simulink model "slexDynamicSchedulingExample"  (R2019b)
settings: Solver=FixedStepAuto  StartTime=0.0  StopTime=1  FixedStep=1  RelTol=1e-3
libraries: simulink x2
settings Model: Creator=The MathWorks, Inc.  LastModifiedBy=bhisma
settings DataIOCC: SaveFormat=Array
settings OptimizationCC: DefaultParameterBehavior=Inlined  PassReuseOutputArgsThreshold=0
settings DebuggingCC: ParameterTunabilityLossMsg=error  ArithmeticOperatorsInVariantConditions=warning
settings SFSimCC: SimUseLocalCustomCode=off  MATLABDynamicMemAlloc=off  CustomCodeUndefinedFunction=UseInterfaceOnly
settings RTWCC: Description=Generic Real-Time Target  GenerateReport=on  RTWUseLocalCustomCode=off  LaunchReport=on
settings CodeAppCC: ForceParamTrailComments=on  OperatorAnnotations=on

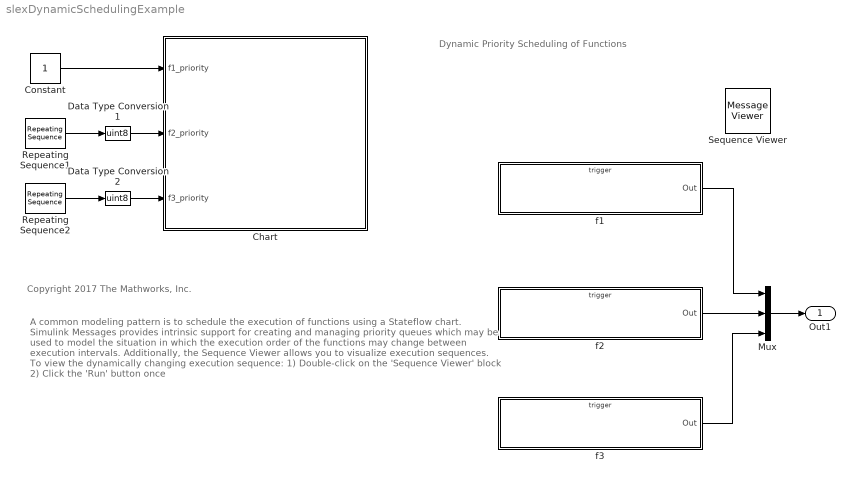
== system slexDynamicSchedulingExample ==
  note: A common modeling pattern is to schedule the execution of functions using a Stateflow chart. Simulink Messages provides intrinsic support for creating and managing priority queues which may be used to model the situation in which the execution order of the functions may change between execution intervals.
      |
      | Additionally, the Sequence Viewer allows you to visualize execution sequences. To view the dynamically changing execution sequence:
      | 1) Double-click on the 'Sequence Viewer' block
      | 2) Click the 'Run' button once
  note: Dynamic Priority Scheduling of Functions
  note: Copyright 2017 The Mathworks, Inc.
  Chart : Stateflow chart  TreatAsAtomicUnit=on
  Constant : Constant  OutDataTypeStr=uint8
  Data Type Conversion1 : DataTypeConversion  OutDataTypeStr=uint8
  Data Type Conversion2 : DataTypeConversion  OutDataTypeStr=uint8
  Mux : Mux  Inputs=3
  Repeating Sequence1 : simulink/Sources/Repeating Sequence  rep_seq_t=[0 1 2]  rep_seq_y=[2 3 2]
  Repeating Sequence2 : simulink/Sources/Repeating Sequence  rep_seq_t=[0 1 2]  rep_seq_y=[3 2 3]
  Sequence Viewer : MessageViewer  History=1000
  f1 : Subsystem  TreatAsAtomicUnit=on
  f2 : Subsystem  TreatAsAtomicUnit=on
  f3 : Subsystem  TreatAsAtomicUnit=on
  Out1 : Outport  VectorParamsAs1DForOutWhenUnconnected=off
  wires:
  Repeating Sequence1/1 -> Data Type Conversion1/1
  Repeating Sequence2/1 -> Data Type Conversion2/1
  Constant/1 -> Chart/1(f1_priority)
  Data Type Conversion1/1 -> Chart/2(f2_priority)
  Data Type Conversion2/1 -> Chart/3(f3_priority)
  f1/1(Out) -> Mux/1
  f3/1(Out) -> Mux/3
  Mux/1 -> Out1/1
  f2/1(Out) -> Mux/2

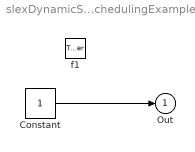
== system slexDynamicSchedulingExample/f1 ==
  f1 : TriggerPort  TriggerType=function-call  IsSimulinkFunction=on  FunctionName=f1  VariantControl=Variant
  Constant : Constant
  Out : Outport  VectorParamsAs1DForOutWhenUnconnected=off
  wires:
  Constant/1 -> Out/1

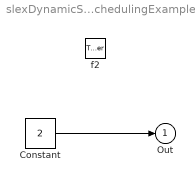
== system slexDynamicSchedulingExample/f2 ==
  f2 : TriggerPort  TriggerType=function-call  IsSimulinkFunction=on  FunctionName=f2  VariantControl=Variant
  Constant : Constant  Value=2
  Out : Outport  VectorParamsAs1DForOutWhenUnconnected=off
  wires:
  Constant/1 -> Out/1

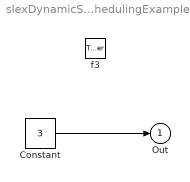
== system slexDynamicSchedulingExample/f3 ==
  f3 : TriggerPort  TriggerType=function-call  IsSimulinkFunction=on  FunctionName=f3  VariantControl=Variant
  Constant : Constant  Value=3
  Out : Outport  VectorParamsAs1DForOutWhenUnconnected=off
  wires:
  Constant/1 -> Out/1

== stateflow chart slexDynamicSchedulingExample/Chart ==
  settings: executeAtInitialization=1
  state fill_queue [parallel]
    settings: executionOrder=1
    note: To add a new function,
        | 1 - Create a new state here
        | 2 - Create a switch case within process function
    state f1 [parallel]
      du: request(1, f1_priority);
      settings: executionOrder=1
    state f2 [parallel]
      du: request(2, f2_priority);
      settings: executionOrder=2
    state f3 [parallel]
      du: request(3, f3_priority);
      settings: executionOrder=3
    state request(function_identifier, function_priority) [function]
      (default) -> (junction 6) : {
          |   pri = bitshift(function_priority, 5);
          |   queue.data = bitor(pri, function_identifier);
          |   send(queue);
          | }
  state process_queue [parallel]
    du: process();
    settings: executionOrder=2
    state process [function]
      (junction 20) -> (junction 24) [order 2]
      (default) -> (junction 20)
      (junction 70) -> (junction 20) : { discard(queue); }
      (junction 58) -> (junction 70)
      (junction 62) -> (junction 70)
      (junction 66) -> (junction 70)
      (junction 81) -> (junction 70)
      (junction 20) -> (junction 25) [order 1] : queue
      (junction 25) -> (junction 28) : {
          |    mask = uint8(bin2dec('11111'));
          |    function_id = bitand(queue.data, mask);
          | }
      (junction 28) -> (junction 57)
      (junction 57) -> (junction 58) [order 1] : [function_id == 1] {f1;}
      (junction 57) -> (junction 61) [order 2]
      (junction 61) -> (junction 62) [order 1] : [function_id == 2] {f2;}
      (junction 61) -> (junction 65) [order 2]
      (junction 65) -> (junction 66) [order 1] : [function_id == 3] {f3;}
      (junction 65) -> (junction 72) [order 2]
      (junction 72) -> (junction 81)
  data: function_identifier function_input uint8; function_priority function_input uint8; queue local; f1_priority input uint8; f2_priority input uint8; f3_priority input uint8
